simulink model "n98tot98reg57neu"  (R2023b)
settings: Solver=VariableStepAuto  StartTime=0.0  StopTime=10.0  RelTol=1e-3
libraries: neural x63
(part 3 of 3)

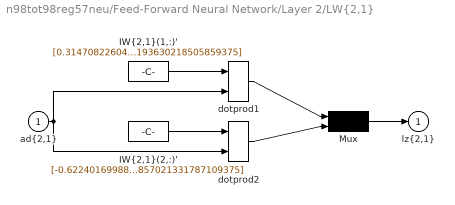
== system n98tot98reg57neu/Feed-Forward Neural Network/Layer 2/LW{2,1} ==
  "ad{2,1}" : Inport  PortDimensions=57
      mask Display: e = 0.06;c1 = [120 230 180]/255;c2 = ([120 230 180]+0)/(256+128);c3 = ([120 230 180]+128)/(256+128);patch([0 1 1 0],[0 0 1 1],c1);patch([0 1 1 1-e 1-e 0+e],[0 0 1 1-e 0+e 0+e],c2);patch([0 0 1 1-e 0+e 0+e],[0 1 1 1-e 1-e 0+e],c3);plot([0 1 1 0 0],[0 0 1 1 0]);
  "IW{2,1}(1,:)'" : Constant  Value=[0.314708226044648375907542003915295936167240142822265625;-0.294686087625244341747787757412879727780818939208984375;-0.192134660175882709953754101661616005003452301025390625;-0.92262035528866859213081852431059814989566802978515625;0.4688111698808883343048137248842976987361907958984375;-1.095590043664996127148469895473681390285491943359375;0.486761718131842047174728804748156107962131500244140625;0.448831403591398558905467552904156036674976348876953125;0.70381709261437974678443652010173536837100982666015625;0.187379720153938500448731474534724839031696319580078125;-0.01123812685505593510215671670948722749017179012298583984375;0.68745585094466921116662661006557755172252655029296875;-0.63725753232719828389463145867921411991119384765625;0.09493829412651048904603356959341908805072307586669921875;0.1551871473607783491477363213562057353556156158447265625;-0.167062135153153545896742571130744181573390960693359375;0.0268075840776443204138690390436750021763145923614501953125;-0.96588300239003699321216345197171904146671295166015625;-1.4051401984263234279382004388025961816310882568359375;-0.055753677592407201168978048144708736799657344818115234375;0.41820281481709742354979653100599534809589385986328125;0.51669261259880638892383331040036864578723907470703125;-0.1267793154429773527791525111751980148255825042724609375;-0.5199619584771941749323787007597275078296661376953125;0.42479040150107960638337090131244622170925140380859375;-0.254226214584103604732234771290677599608898162841796875;0.101011071529465812357528875509160570800304412841796875;0.3694710281678201813093664895859546959400177001953125;-0.95881509200480985466441552489413879811763763427734375;0.49025519141012219304087693672045134007930755615234375;0.26020636652179851555644063409999944269657135009765625;-0.270252416063623324138376347036683000624179840087890625;-0.30044681010318396996439105350873433053493499755859375;-0.25832065503474443968201512689120136201381683349609375;0.54805354694859798048156562799704261124134063720703125;-0.12319716258758195426281645268318243324756622314453125;1.272522835964362553085038598510436713695526123046875;-0.54251828710713834169609981472603976726531982421875;0.28781359819066698602085807578987441956996917724609375;0.43997570178121125916703704206156544387340545654296875;0.783961157676562603313641375279985368251800537109375;-0.5407643557439436587941372636123560369014739990234375;0.09672278407687472101539327695718384347856044769287109375;-0.82467231078483826944847123741055838763713836669921875;-0.2144768839952212735600056703333393670618534088134765625;-0.88972040353890491370947302129934541881084442138671875;-3.04292029362801041969532889197580516338348388671875;-0.13786343394404843021305850925273261964321136474609375;0.288889316805307772018096557076205499470233917236328125;1.046720223143054351311320715467445552349090576171875;-0.7391460152023598961790185057907365262508392333984375;0.92419761569726954775205740588717162609100341796875;-0.2187601892939461667442202497113612480461597442626953125;-0.6341221805653987075857003219425678253173828125;0.41314393086403666810468848780146799981594085693359375;-0.487595671484026327302530035012750886380672454833984375;-1.538315111603009821550358537933789193630218505859375]
      mask Display: e = 0.06;c1 = [120 150 230]/255;c2 = ([120 150 230]+0)/383;c3 = ([120 150 230]+128)/383;patch([0 1 1 0],[0 0 1 1],c1);patch([0 1 1 1-e 1-e 0+e],[0 0 1 1-e 0+e 0+e],c2);patch([0 0 1 1-e 0+e 0+e],[0 1 1 1-e 1-e 0+e],c3);plot([0 1 1 0 0],[0 0 1 1 0]);disp('weights');
  "IW{2,1}(2,:)'" : Constant  Value=[-0.62240169988661675493091252064914442598819732666015625;0.297659352616439332184228305777651257812976837158203125;0.5590509920651645092704029593733139336109161376953125;-0.51980503949221457116180999946664087474346160888671875;0.305080343278699928077912773005664348602294921875;-0.1906121016839554538346845902196946553885936737060546875;-0.388819356678638594626562507983180694282054901123046875;0.99899991791156950160512906222720630466938018798828125;0.59132290791277475339171587620512582361698150634765625;-0.195284409726231789061756671799230389297008514404296875;-0.1799942407769452301646850855831871740520000457763671875;-0.277178880329822463490785366957425139844417572021484375;0.21677677761771663167422730111866258084774017333984375;0.45609818696839543594734323050943203270435333251953125;-0.11480906696614474882256473620145698077976703643798828125;-0.5480390980209914886245314846746623516082763671875;-0.0619245811847038141184640380743076093494892120361328125;-0.27807261297143048839330958799109794199466705322265625;0.5070256987067740528374315545079298317432403564453125;0.6802261371729716454836989214527420699596405029296875;-0.38977865990637550197561722598038613796234130859375;-0.25085291239600249202368331680190749466419219970703125;-0.3446233703577676887874758904217742383480072021484375;0.189494624767892194672214145612088032066822052001953125;-0.0735322839353736157352869895476032979786396026611328125;-0.00732921642620550095603704221502994187176227569580078125;-0.82229904555818833511438015193562023341655731201171875;0.028772351282397724825390383784906589426100254058837890625;-0.9295612827231891639456762277404777705669403076171875;-0.344354739444726998254253658160450868308544158935546875;0.315003152981325029724501973760197870433330535888671875;-0.54275024947517402917895878999843262135982513427734375;-0.2190536303888607483347783499993965961039066314697265625;-0.98506087360740857139518311669235117733478546142578125;0.66452258995670543395561935540172271430492401123046875;0.7059530604308574819327759541920386254787445068359375;-0.65436576453843098288842838883283548057079315185546875;0.2492419570367940817590124424896202981472015380859375;1.0063646375063213245226734215975739061832427978515625;-0.0149996194721860598431106836869730614125728607177734375;1.0749448971504718119973631473840214312076568603515625;-0.66399361980437221486539556281059049069881439208984375;-0.54472977068269090583640945624210871756076812744140625;-0.340045747638266615542335102873039431869983673095703125;-0.254496410453752541780403362281504087150096893310546875;0.00938084139282686739480521254108680295757949352264404296875;0.10145524560216680198809768853607238270342350006103515625;-0.406331250181566960844037339484202675521373748779296875;-0.17213059708636613276411253536934964358806610107421875;0.1605952273253431761279585998636321164667606353759765625;-0.5789809913520913564610737012117169797420501708984375;0.1375647743787366816814454750783625058829784393310546875;0.054026746582682784458828706419808440841734409332275390625;-0.6934918717140383659369717861409299075603485107421875;-0.43314038439945601322023094326141290366649627685546875;-0.492323691757734327456574874304351396858692169189453125;-0.295120972702875794535515296956873498857021331787109375]
      mask Display: e = 0.06;c1 = [120 150 230]/255;c2 = ([120 150 230]+0)/383;c3 = ([120 150 230]+128)/383;patch([0 1 1 0],[0 0 1 1],c1);patch([0 1 1 1-e 1-e 0+e],[0 0 1 1-e 0+e 0+e],c2);patch([0 0 1 1-e 0+e 0+e],[0 1 1 1-e 1-e 0+e],c3);plot([0 1 1 0 0],[0 0 1 1 0]);disp('weights');
  Mux : Mux  Inputs=2
      mask Display: e = 0.06;c1 = [120 150 230]/255;c2 = ([120 150 230]+0)/383;c3 = ([120 150 230]+128)/383;patch([0 1 1 0],[0 0 1 1],c1);patch([0 1 1 1-e 1-e 0+e],[0 0 1 1-e 0+e 0+e],c2);patch([0 0 1 1-e 0+e 0+e],[0 1 1 1-e 1-e 0+e],c3);plot([0 1 1 0 0],[0 0 1 1 0]);disp('Mux');
  dotprod1 : neural/Weight Functions/dotprod
  dotprod2 : neural/Weight Functions/dotprod
  "lz{2,1}" : Outport
      mask Display: e = 0.06;c1 = [120 230 180]/255;c2 = ([120 230 180]+0)/(256+128);c3 = ([120 230 180]+128)/(256+128);patch([0 1 1 0],[0 0 1 1],c1);patch([0 1 1 1-e 1-e 0+e],[0 0 1 1-e 0+e 0+e],c2);patch([0 0 1 1-e 0+e 0+e],[0 1 1 1-e 1-e 0+e],c3);plot([0 1 1 0 0],[0 0 1 1 0]);
  wires:
  "IW{2,1}(1,:)'"/1 -> dotprod1/1
  "ad{2,1}"/1 -> dotprod1/2, dotprod2/2
  dotprod1/1 -> Mux/1
  "IW{2,1}(2,:)'"/1 -> dotprod2/1
  dotprod2/1 -> Mux/2
  Mux/1 -> "lz{2,1}"/1
